simulink model "computed_torque_controller"  (R2019b)
settings: Solver=VariableStepAuto  StartTime=0.0  StopTime=10.0  RelTol=1e-3
undefined symbols (not defined in the file): Kd, Kp, m
settings Model: Creator=logan  LastModifiedBy=logan
settings DataIOCC: ReturnWorkspaceOutputs=off
settings DebuggingCC: ArithmeticOperatorsInVariantConditions=warning
settings SFSimCC: CustomCodeUndefinedFunction=UseInterfaceOnly

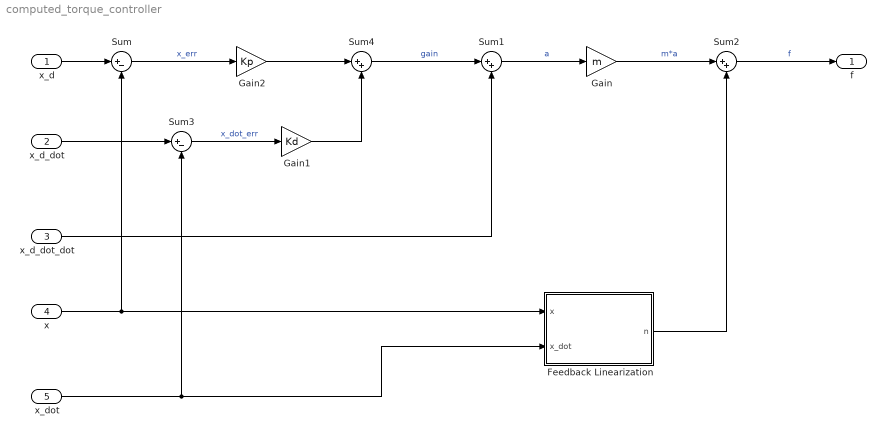
== system computed_torque_controller ==
  x_d : Inport
  "x_d_dot " : Inport  Port=2
  "x_d_dot_dot " : Inport  Port=3
  "x " : Inport  Port=4
  x_dot : Inport  Port=5
  Feedback Linearization : MATLAB Function  TreatAsAtomicUnit=on
  Gain : Gain  Gain=m
  Gain1 : Gain  Gain=Kd
  Gain2 : Gain  Gain=Kp
  Sum : Sum  Inputs=|+-
  Sum1 : Sum  Inputs=|++
  Sum2 : Sum  Inputs=|++
  Sum3 : Sum  Inputs=|+-
  Sum4 : Sum  Inputs=|++
  f : Outport
  wires:
  "x "/1 -> Feedback Linearization/1(x), Sum/2
  x_d/1 -> Sum/1
  "x_d_dot_dot "/1 -> Sum1/2
  Sum1/1 -> Gain/1  "a"
  Gain/1 -> Sum2/1  "m*a"
  Feedback Linearization/1(n) -> Sum2/2
  x_dot/1 -> Sum3/2, Feedback Linearization/2(x_dot)
  Sum2/1 -> f/1  "f"
  "x_d_dot "/1 -> Sum3/1
  Sum3/1 -> Gain1/1  "x_dot_err"
  Gain1/1 -> Sum4/2
  Gain2/1 -> Sum4/1
  Sum4/1 -> Sum1/1  "gain"
  Sum/1 -> Gain2/1  "x_err"

== matlab function computed_torque_controller/Feedback Linearization ==
  data: x input; n output; x_dot input
function n = fcn(x, x_dot)

n = 2*x_dot;
